simulink model "Battery_charge_discharge_FSBB_DCDC"  (R2022b)
settings: Solver=ode23tb  StartTime=0.0  StopTime=1.5  RelTol=1e-3  EnableMultiTasking=on
values from neighbouring files (symbols this model uses):
  time_step = 1 / wave_freq    (= 1.11111111111e-05)    [Battery_charge_discharge_FSBB_param_init.m]
undefined symbols (not defined in the file or in its folder): Ion, Lithium
libraries: spsTriangleGeneratorLib x13, spsSeriesRLCBranchLib x9, slpidlib x9, spsVoltageMeasurementLib x5, spsCurrentMeasurementLib x4, spsIGBTDiodeLib x4, spsBatteryLib x2, spsIdealSwitchLib x2, spsDCVoltageSourceLib x2, spsControlledVoltageSourceLib x1, spspowerguiLib x1
(part 1 of 2)
settings Model: Creator=Lei  LastModifiedBy=Loki
settings SolverCC: AlgebraicLoopSolver=TrustRegion
settings DataIOCC: LimitDataPoints=on  SaveFormat=Array  ReturnWorkspaceOutputs=off
settings OptimizationCC: LifeSpan=inf
settings DebuggingCC: SolverPrmCheckMsg=warning  UnconnectedInputMsg=warning  UnconnectedOutputMsg=warning  UnconnectedLineMsg=warning  SFUnexpectedBacktrackingDiag=warning  SFNoUnconditionalDefaultTransitionDiag=warning  SFExecutionAtInitializationDiag=none  SFMachineParentedDataDiag=warning  ArithmeticOperatorsInVariantConditions=warning
settings HardwareCC: ProdBitPerPointer=32  ProdBitPerSizeT=32  ProdBitPerPtrDiffT=32  ProdLargestAtomicFloat=None  ProdIntDivRoundTo=Undefined  ProdEndianess=Unspecified  ProdWordSize=32  ProdHWDeviceType=32-bit Generic
settings ModelReferenceCC: EnableRefExpFcnMdlSchedulingChecks=on  PropagateSignalLabelsOutOfModel=off
settings SFSimCC: SimUseLocalCustomCode=off  CustomCodeUndefinedFunction=UseInterfaceOnly
settings RTWCC: RTWUseLocalCustomCode=off
settings CodeAppCC: StateflowObjectComments=on
settings GRTTargetCC: TargetLangStandard=C89/C90 (ANSI)
settings ConfigComp: CovMetricSettings=dw  CovSaveCumulativeToWorkspaceVar=on  CovSaveSingleToWorkspaceVar=on  CovExternalEMLEnable=off  CovSFcnEnable=off
settings SimscapeCC: SimscapeNormalizeSystem=off

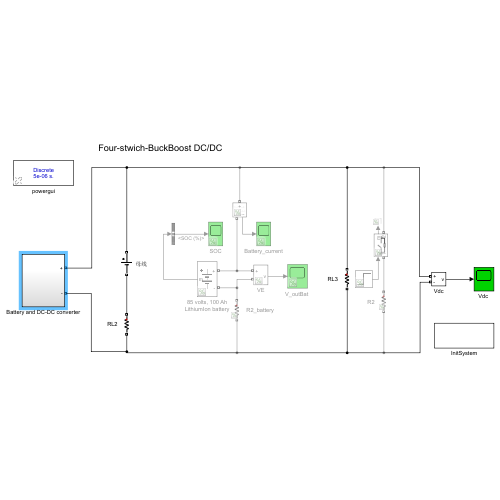
[thumbnail: Simulink's stored preview of the top-level diagram]
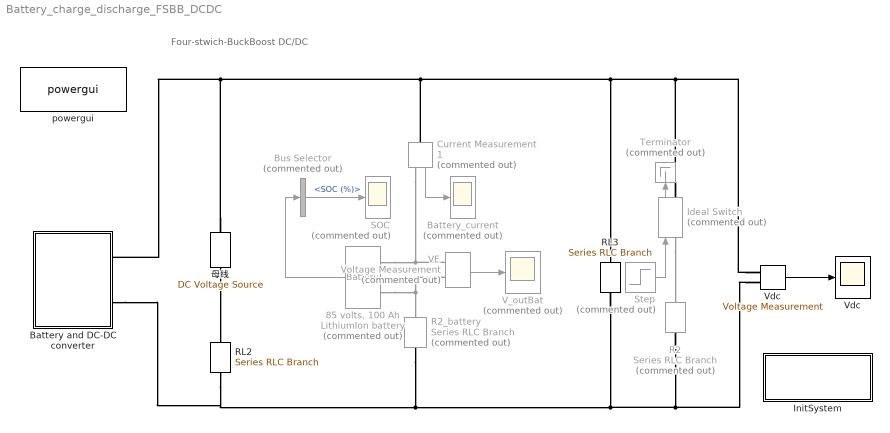
== system Battery_charge_discharge_FSBB_DCDC ==
  note: Four-stwich-BuckBoost DC/DC
  "85 volts, 100 Ah LithiumIon battery " : spsBatteryLib/Battery  Commented=on  BatType=Lithium-Ion  ShowTempParam=off  ThermalPreset=no  ShowAgeParam=off  NomV=85  NomQ=100  SOC=90  Batt_Tr=30  PresetModel=off  MaxQ=107.6923  MinV=83.2  FullV=115.2  Dis_rate=20  R=0.0085  Normal_OP=96.1538  expZone="[92.2034           20]"  current=[6.5 13 32.5]  Units=Time  Tci=20  NomT=20  T2=-30  MaxQ2=4.8  FullV2=7.1  Normal_OP2=5.655  expZone2="[6.58           1]"  Rca=0.6  ti=2000  Dp=0  Neq0=0  Tsim=1e6  Ta1=25  Qeol=5.4*0.9  Reol=0.013333*1.2  Char_age=[2.3478, 3]  Dis_age=[2.3478, 10]  N1=1500  N2=10500  N3=1000  N4=1400  Ta2=45  N5=950
      settings: LibrarySourceBlock=electricdrivelib/Extra Sources/Battery
  Battery and DC-DC converter : Subsystem
  Battery_current : Scope  Commented=on
  Bus Selector : BusSelector  Commented=on  OutputSignals=SOC (%)
  Current Measurement1 : spsCurrentMeasurementLib/Current Measurement  Commented=on  PhasorSimulation=off  OutputType=Complex  PSBequivalent=0
  Ideal Switch : spsIdealSwitchLib/Ideal Switch  Commented=on  Ron=0.001  Lon=0  IC=0  Rs=1e5  Cs=inf  Measurements=on
  InitSystem : Subsystem
      settings: OpenFcn=Battery_charge_discharge_FSBB_param_init
  R2 : spsSeriesRLCBranchLib/Series RLC Branch  Commented=on  LConnTagsString=__new0  RConnTagsString=__new0  BranchType=R  Resistance=6  Inductance=1e-3  SetiL0=off  InitialCurrent=0  Capacitance=1e-6  Setx0=off  InitialVoltage=0  Measurements=None
  R2_battery : spsSeriesRLCBranchLib/Series RLC Branch  Commented=on  LConnTagsString=__new0  RConnTagsString=__new0  BranchType=R  Resistance=0.1  Inductance=1e-3  SetiL0=off  InitialCurrent=0  Capacitance=1440e-6  Setx0=off  InitialVoltage=80  Measurements=None
  RL2 : spsSeriesRLCBranchLib/Series RLC Branch  LConnTagsString=__new0  RConnTagsString=__new0  BranchType=R  Resistance=0.1  Inductance=1e-3  SetiL0=off  InitialCurrent=0  Capacitance=1e-6  Setx0=off  InitialVoltage=0  Measurements=None
  RL3 : spsSeriesRLCBranchLib/Series RLC Branch  LConnTagsString=__new0  RConnTagsString=__new0  BranchType=R  Resistance=6  Inductance=1e-3  SetiL0=off  InitialCurrent=0  Capacitance=1e-6  Setx0=off  InitialVoltage=0  Measurements=None
  SOC : Scope  Commented=on
  Step : Step  Commented=on  Time=0.3  After=3  SampleTime=0
  Terminator : Terminator  Commented=on
  VE : spsVoltageMeasurementLib/Voltage Measurement  Commented=on  PhasorSimulation=off  OutputType=Complex  PSBequivalent=0
  "V_outBat " : Scope  Commented=on
  Vdc : spsVoltageMeasurementLib/Voltage Measurement  PhasorSimulation=off  OutputType=Complex  PSBequivalent=0
  "Vdc " : Scope
  powergui : spspowerguiLib/powergui  Priority=1  SimulationMode=Discrete  SampleTime=5e-6  frequency=60  Iterations=50  frequencyindice=0  Pbase=100e6  ErrMax=1e-4  UnitsV=kV  UnitsW=MW  buscounter=0  FunctionMessages=off  echomessages=off  EnableUseOfTLC=off  CurrentSourceSwitches=off  DisableSnubberDevices=off  DisableRonSwitches=off  DisableVfSwitches=off  DisplayEquations=off  AutomaticDiscreteSolvers=off  SolverType=Tustin/Backward Euler (TBE)  Interpol=off  ExternalGateDelay=off  methode=off  Ts=100  x0status=blocks  SPID=off  SwTol=0  HookPort=off  NonlinearTolerance=1e-4  nMaxIteration=100  ContinueOnMaxIteration=off  RestoreLinks=warning  ResistiveCurrentMeasurement=off  Frange=[0:2:500]  Ylog=off  Xlog=on  ShowGrid=off  save=off  variable=ZData  structure=0  ZoomFFT=off  StartTime=0.0  cycles=1  DisplayStyle=1  fundamental=60  FreqAxis=off  MaxFrequency=1000  frequencyindicesteady=1  RmsSteady=1  display=off
  "母线  " : spsDCVoltageSourceLib/DC Voltage Source  Amplitude=104  Measurements=None
  wires:
  Vdc/1 -> "Vdc "/1
  Step/1 -> Ideal Switch/1
  Ideal Switch/1 -> Terminator/1
  Bus Selector/1 -> SOC/1  "<SOC (%)>"
  "85 volts, 100 Ah LithiumIon battery "/1 -> Bus Selector/1
  Current Measurement1/1 -> Battery_current/1
  VE/1 -> "V_outBat "/1
  connections:
  Vdc/LConn1 -- Ideal Switch/RConn1 -- Current Measurement1/LConn1 -- "母线  "/RConn1 -- Battery and DC-DC converter/RConn1 -- RL3/LConn1
  Vdc/LConn2 -- R2/RConn1 -- RL3/RConn1 -- RL2/RConn1 -- Battery and DC-DC converter/RConn2 -- R2_battery/RConn1
  "母线  "/LConn1 -- RL2/LConn1
  Ideal Switch/LConn1 -- R2/LConn1
  VE/LConn2 -- "85 volts, 100 Ah LithiumIon battery "/LConn2 -- R2_battery/LConn1
  VE/LConn1 -- Current Measurement1/RConn1 -- "85 volts, 100 Ah LithiumIon battery "/LConn1

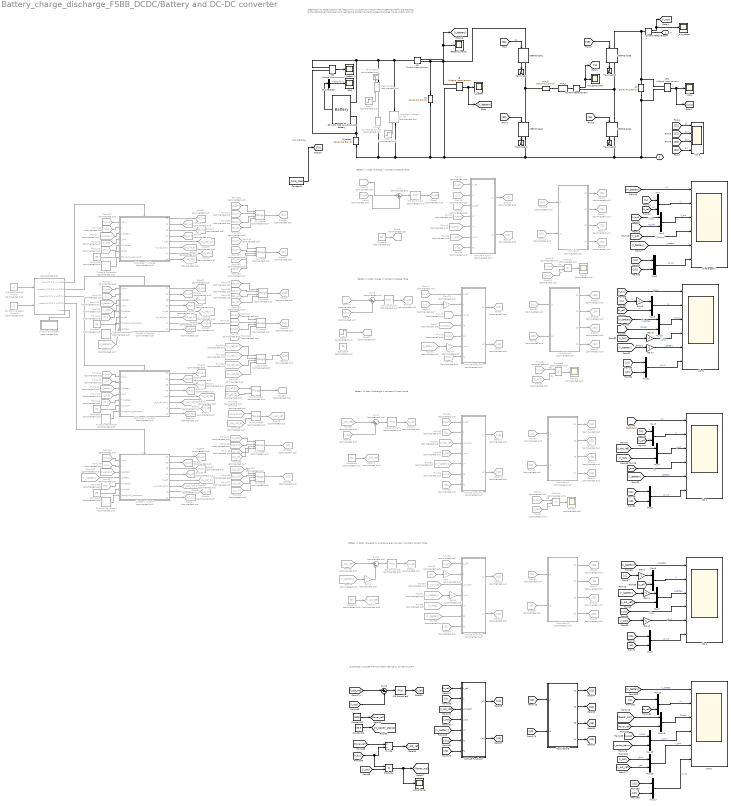
== system Battery_charge_discharge_FSBB_DCDC/Battery and DC-DC converter ==
  note: Discharge in Constant Power Mode: realize by constant current
  note: Battery in dcdc , charged by outside energy source in constant Current Mode
  note: Battery in dcdc ,discharge in constant Current Mode
  note: Battery in dcdc, dicharge in constant Voltage Mode
  note: 和开关频率同步
  note: FSBB Passivity Based Control
      | ref: https://www.youtube.com/watch?v=5YT7cERlMrg
      | Modify the topology to the Gosspower hardware's
      | and realize the constant current/voltage discharge mode.
      | Author LokiXun
  note: Battery in dcdc, charge in constant Voltage Mode
  "85 volts, 100 Ah LithiumIon battery " : spsBatteryLib/Battery  BatType=Lithium-Ion  ShowTempParam=off  ThermalPreset=no  ShowAgeParam=off  NomV=85  NomQ=100  SOC=80  Batt_Tr=30  PresetModel=off  MaxQ=107.6923  MinV=83.2  FullV=115.2  Dis_rate=20  R=0.0085  Normal_OP=96.1538  expZone="[92.2034           20]"  current=[6.5 13 32.5]  Units=Time  Tci=20  NomT=20  T2=-30  MaxQ2=4.8  FullV2=7.1  Normal_OP2=5.655  expZone2="[6.58           1]"  Rca=0.6  ti=2000  Dp=0  Neq0=0  Tsim=1e6  Ta1=25  Qeol=5.4*0.9  Reol=0.013333*1.2  Char_age=[2.3478, 3]  Dis_age=[2.3478, 10]  N1=1500  N2=10500  N3=1000  N4=1400  Ta2=45  N5=950
      settings: LibrarySourceBlock=electricdrivelib/Extra Sources/Battery
  ActualPower : Scope
  BatteryCurrent1 : Scope
  Bus Selector : BusSelector  OutputSignals=SOC (%)
  C1 : spsSeriesRLCBranchLib/Series RLC Branch  LConnTagsString=__new0  RConnTagsString=__new0  BranchType=C  Resistance=0.01  Inductance=1e-3  SetiL0=off  InitialCurrent=0  Capacitance=1440e-6  Setx0=off  InitialVoltage=80  Measurements=None
  C2 : spsSeriesRLCBranchLib/Series RLC Branch  LConnTagsString=__new0  RConnTagsString=__new0  BranchType=C  Resistance=5  Inductance=1e-3  SetiL0=off  InitialCurrent=0  Capacitance=1440e-6  Setx0=off  InitialVoltage=80  Measurements=None
  Charge + Current : Subsystem  Commented=on  TreatAsAtomicUnit=on
  Charge + Voltage : Subsystem  Commented=on  TreatAsAtomicUnit=on
  Charge/Discharge Mode : Constant  Commented=on  Value=0
  Constant{,4,6..7} (4 alike) : Constant  Commented=on  Value=96
  Constant Voltage / Current : Constant  Commented=on
  Constant1 : Constant  Value=time_step
  Constant10 : Constant  Value=3000
  Constant11 : Constant  Value=103.5
  Constant2 : Constant  Commented=on  Value=30
  Constant3 : Constant  Commented=on  Value=29
  Constant8 : Constant  Commented=on  Value=29
  Constant9 : Constant  Commented=on  Value=29
  Controlled Voltage Source : spsControlledVoltageSourceLib/Controlled Voltage Source  Commented=on  Initialize=on  Source_Type=DC  Amplitude=103  Phase=0  Frequency=0  Measurements=None
  Current Measurement : spsCurrentMeasurementLib/Current Measurement  PhasorSimulation=off  OutputType=Complex  PSBequivalent=0
  Current Measurement1 : spsCurrentMeasurementLib/Current Measurement  PhasorSimulation=off  OutputType=Complex  PSBequivalent=0
  Discharge + Current : Subsystem  Commented=on  TreatAsAtomicUnit=on
  Discharge + Voltage : Subsystem  Commented=on  TreatAsAtomicUnit=on
  Discharge+V : Scope  NumInputPorts=6
  Divide : Product  Inputs=*/
  From{10,24,30,32,116,121,143,156} (8 alike) : From  Commented=on  GotoTag=iL
  From{11..12,70,75} (4 alike) : From  Commented=on  GotoTag=VC_ref
  From{8,13,28,41,52..53,76,92,94,115,120,142,155} (13 alike) : From  Commented=on  GotoTag=V_bus
  From{14,33,59,77,117,122,144,157} (8 alike) : From  Commented=on  GotoTag=V_battery
  From{29,31,42,55,88,96,118,123,145} (9 alike) : From  Commented=on  GotoTag=i_out
  From{18,35,54,78,119,124,146,159} (8 alike) : From  Commented=on  GotoTag=Ts
  From125 : From  Commented=on  GotoTag=S1_DV
  From126 : From  Commented=on  GotoTag=S2_DV
  From127 : From  Commented=on  GotoTag=S1_CV
  From128 : From  Commented=on  GotoTag=S2_CV
  From129 : From  Commented=on  GotoTag=S3_DV
  From130 : From  Commented=on  GotoTag=S3_CV
  From131 : From  Commented=on  GotoTag=S4_CV
  From132 : From  Commented=on  GotoTag=S4_DV
  From133 : From  Commented=on  GotoTag=iL_ref_CV
  From134 : From  Commented=on  GotoTag=iL_ref_DV
  From135 : From  Commented=on  GotoTag=VC_ref_CV
  From136 : From  Commented=on  GotoTag=VC_ref_DV
  From137 : From  Commented=on  GotoTag=u1_DV
  From138 : From  Commented=on  GotoTag=u1_CV
  From139 : From  Commented=on  GotoTag=u2_DV
  From140 : From  Commented=on  GotoTag=u2_CV
  From{34,74,95,141,160} (5 alike) : From  Commented=on  GotoTag=i_battery
  From147 : From  Commented=on  GotoTag=u2_DI
  From148 : From  Commented=on  GotoTag=u1_DI
  From149 : From  Commented=on  GotoTag=i_out_ref_DI
  From150 : From  Commented=on  GotoTag=iL_ref_DI
  From151 : From  Commented=on  GotoTag=S4_DI
  From152 : From  Commented=on  GotoTag=S3_DI
  From153 : From  Commented=on  GotoTag=S2_DI
  From154 : From  Commented=on  GotoTag=S1_DI
  From158 : From  Commented=on  GotoTag=i_out_ref_CI
  From{16,39,61,80} (4 alike) : From  Commented=on  GotoTag=u1
  From161 : From  Commented=on  GotoTag=S1_CI
  From162 : From  Commented=on  GotoTag=S2_CI
  From163 : From  Commented=on  GotoTag=S3_CI
  From164 : From  Commented=on  GotoTag=S4_CI
  From165 : From  Commented=on  GotoTag=iL_ref_CI
  From166 : From  Commented=on  GotoTag=u1_CI
  From167 : From  Commented=on  GotoTag=u2_CI
  From{17,40,62,81} (4 alike) : From  Commented=on  GotoTag=u2
  From{9,36,56,79} (4 alike) : From  Commented=on  GotoTag=iL_ref
  From{37..38,57..58} (4 alike) : From  Commented=on  GotoTag=i_out_ref
  Gain{,2..3,6,10} (5 alike) : Gain  Commented=on  Gain=-1
  Gain{1,4..5,7..9} (6 alike) : Gain  Gain=-1
  Goto{10,21,28..29,58} (5 alike) : Goto  Commented=on  GotoTag=S4
  Goto{11,22,30,33,56} (5 alike) : Goto  Commented=on  GotoTag=S2
  Goto{6,12,15,17,61} (5 alike) : Goto  Commented=on  GotoTag=u1
  Goto{7,14,18,25,62} (5 alike) : Goto  Commented=on  GotoTag=u2
  Goto19 : Goto  Commented=on  GotoTag=i_out_ref
  Goto{2,20,27,36,60} (5 alike) : Goto  Commented=on  GotoTag=iL_ref
  Goto{8,23,31,40,59} (5 alike) : Goto  Commented=on  GotoTag=S1
  Goto{9,24,32,41,57} (5 alike) : Goto  Commented=on  GotoTag=S3
  Goto26 : Goto  Commented=on  GotoTag=i_out_ref
  Goto37 : Goto  Commented=on  GotoTag=VC_ref
  Goto47 : Goto  Commented=on  GotoTag=VC_ref_DV
  Goto48 : Goto  Commented=on  GotoTag=S2_DV
  Goto49 : Goto  Commented=on  GotoTag=S3_DV
  Goto5 : Goto  Commented=on  GotoTag=VC_ref
  Goto50 : Goto  Commented=on  GotoTag=S4_DV
  Goto51 : Goto  Commented=on  GotoTag=S1_DV
  Goto52 : Goto  Commented=on  GotoTag=iL_ref_DV
  Goto53 : Goto  Commented=on  GotoTag=u1_DV
  Goto54 : Goto  Commented=on  GotoTag=u2_DV
  Goto55 : Goto  Commented=on  GotoTag=VC_ref
  Goto63 : Goto  Commented=on  GotoTag=VC_ref_CV
  Goto64 : Goto  Commented=on  GotoTag=S2_CV
  Goto65 : Goto  Commented=on  GotoTag=S3_CV
  Goto66 : Goto  Commented=on  GotoTag=S4_CV
  Goto67 : Goto  Commented=on  GotoTag=S1_CV
  Goto68 : Goto  Commented=on  GotoTag=iL_ref_CV
  Goto69 : Goto  Commented=on  GotoTag=u1_CV
  Goto70 : Goto  Commented=on  GotoTag=u2_CV
  Goto71 : Goto  Commented=on  GotoTag=i_out_ref_DI
  Goto72 : Goto  Commented=on  GotoTag=S2_DI
  Goto73 : Goto  Commented=on  GotoTag=S3_DI
  Goto74 : Goto  Commented=on  GotoTag=S4_DI
  Goto75 : Goto  Commented=on  GotoTag=S1_DI
  Goto76 : Goto  Commented=on  GotoTag=iL_ref_DI
  Goto77 : Goto  Commented=on  GotoTag=u1_DI
  Goto78 : Goto  Commented=on  GotoTag=u2_DI
  Goto79 : Goto  Commented=on  GotoTag=i_out_ref
  Goto80 : Goto  Commented=on  GotoTag=i_out_ref_CI
  Goto81 : Goto  Commented=on  GotoTag=S2_CI
  Goto82 : Goto  Commented=on  GotoTag=S3_CI
  Goto83 : Goto  Commented=on  GotoTag=S4_CI
  Goto84 : Goto  Commented=on  GotoTag=S1_CI
  Goto85 : Goto  Commented=on  GotoTag=iL_ref_CI
  Goto86 : Goto  Commented=on  GotoTag=u1_CI
  Goto87 : Goto  Commented=on  GotoTag=u2_CI
  IGBT/Diode{1..4} (4 alike) : spsIGBTDiodeLib/IGBT//Diode  Ron=1e-3  Rs=1e5  Cs=inf  Measurements=on
  IL6 : spsCurrentMeasurementLib/Current Measurement  PhasorSimulation=off  OutputType=Complex  PSBequivalent=0
  I_bus_scope : Scope
  Ideal Switch : spsIdealSwitchLib/Ideal Switch  Commented=on  Ron=0.001  Lon=0  IC=0  Rs=1e5  Cs=inf  Measurements=on
  If : If  Commented=on  NumInputs=2  IfExpression=u1 == 1 & u2 ==0  ElseIfExpressions=u1 == 0 & u2 ==0, u1==1 & u2==1, u1==0 & u2==1
  If Action Subsystem : Subsystem  Commented=on  TreatAsAtomicUnit=on
  InductorCurrent : Scope
  MATLAB Function : MATLAB Function  Commented=on  TreatAsAtomicUnit=on
  MATLAB Function1 : MATLAB Function  Commented=on  TreatAsAtomicUnit=on
  MATLAB Function2 : MATLAB Function  Commented=on  TreatAsAtomicUnit=on
  MATLAB Function3 : MATLAB Function  Commented=on  TreatAsAtomicUnit=on
  MATLAB Function5 : MATLAB Function  TreatAsAtomicUnit=on
  Modulation : Subsystem  Commented=on
  Modulation1 : Subsystem  Commented=on
  Modulation2 : Subsystem  Commented=on
  Modulation3 : Subsystem  Commented=on
  Modulation5 : Subsystem
  Mux{,1..11,15..19} (17 alike) : Mux  Inputs=2
  PID Controller{1..4} (4 alike) : slpidlib/PID Controller  Commented=on  Controller=PI  Form=Parallel  TimeDomain=Continuous-time  UseExternalTs=off  SampleTime=-1  IntegratorMethod=Forward Euler  FilterMethod=Forward Euler  ControllerParametersSource=internal  P=15  I=1000  UseKiTs=on  D=0  N=100  UseFilter=on  TunerSelectOption=Transfer Function Based (PID Tuner App)  InitialConditionSource=internal  InitialConditionForIntegrator=0  InitialConditionForFilter=0  DifferentiatorICPrevScaledInput=0  ExternalReset=none  TrackingMode=off  Kt=1  LimitOutput=on  SatLimitsSource=internal  UpperSaturationLimit=50  LowerSaturationLimit=-10  LinearizeAsGain=on  AntiWindupMode=none  Kb=1  LimitIntegrator=off  UpperIntegratorSaturationLimit=inf  LowerIntegratorSaturationLimit=-inf  POutMin=[]  POutMax=[]  IOutMin=[]  IOutMax=[]  DOutMin=[]  DOutMax=[]  NOutMin=[]  NOutMax=[]  SumOutMin=[]  SumOutMax=[]  SaturationOutMin=[]  SaturationOutMax=[]  PParamMin=[]  PParamMax=[]  IParamMin=[]  IParamMax=[]  DParamMin=[]  DParamMax=[]  NParamMin=[]  NParamMax=[]  KbParamMin=[]  KbParamMax=[]  KtParamMin=[]  KtParamMax=[]  KbOutMin=[]  KbOutMax=[]  KtOutMin=[]  KtOutMax=[]  IntegratorOutMin=[]  IntegratorOutMax=[]  FilterOutMin=[]  FilterOutMax=[]  SumI1OutMin=[]  SumI1OutMax=[]  SumI2OutMin=[]  SumI2OutMax=[]  SumI3OutMin=[]  SumI3OutMax=[]  SumI4OutMin=[]  SumI4OutMax=[]  SumDOutMin=[]  SumDOutMax=[]  DifferentiatorOutMin=[]  DifferentiatorOutMax=[]  FilterDiffOutCoefMin=[]  FilterDiffOutCoefMax=[]  ReciprocalOutMin=[]  ReciprocalOutMax=[]  SumDenOutMin=[]  SumDenOutMax=[]  SumNumOutMin=[]  SumNumOutMax=[]  DivideOutMin=[]  DivideOutMax=[]  UdiffTsProdOutMin=[]  UdiffTsProdOutMax=[]  NTsProdOutMin=[]  NTsProdOutMax=[]  UintegralTsProdOutMin=[]  UintegralTsProdOutMax=[]  UngainTsProdOutMin=[]  UngainTsProdOutMax=[]  ClampingZeroOutDataTypeStr=Inherit: Inherit via back propagation  ClampingZeroOutMin=[]  ClampingZeroOutMax=[]  FilterDenConstantOutDataTypeStr=Inherit: Inherit via back propagation  FilterDenConstantOutMin=[]  FilterDenConstantOutMax=[]  PCopyOutDataTypeStr=Inherit: Inherit via back propagation  PCopyOutMin=[]  PCopyOutMax=[]  NCopyOutDataTypeStr=Inherit: Inherit via back propagation  NCopyOutMin=[]  NCopyOutMax=[]  IntegratorContinuousStateAttributes=''  IntegratorStateMustResolveToSignalObject=off  IntegratorRTWStateStorageClass=Auto  FilterContinuousStateAttributes=''  FilterStateMustResolveToSignalObject=off  FilterRTWStateStorageClass=Auto  ParallelPVariant=InternalParameters  IdealPVariant=Disabled  IVariant=InternalParameters  DVariant=Disabled  IntegratorVariant=Continuous  SatVariant=Enabled  AWVariant=Passthrough  PCopyVariant=Disabled  TRVariant=Disabled  FdbkBlocksVariant=Forward  IdealPFdbkVariant=Disabled  SatFdbkVariant=Disabled  DerivativeFilterVariant=Disabled  NVariant=Disabled  NCopyVariant=Disabled_SignalSpec  FilterICVariant=Disabled  IntegratorICVariant=InternalICs  ExternalResetVariant=Disabled  TRSumVariant=Passthrough  SumFdbkVariant=Disabled  SumVariant=Sum_PI  TsampFilterVariant=InternalTs  TsampNgainVariant=Passthrough  TsampIntegralVariant=Passthrough  ExternalSaturationOutDataTypeStr=Inherit: Same as second input
  PID Controller6 : slpidlib/PID Controller  Controller=PI  Form=Parallel  TimeDomain=Continuous-time  UseExternalTs=off  SampleTime=-1  IntegratorMethod=Forward Euler  FilterMethod=Forward Euler  ControllerParametersSource=internal  P=15  I=1000  UseKiTs=on  D=0  N=100  UseFilter=on  TunerSelectOption=Transfer Function Based (PID Tuner App)  InitialConditionSource=internal  InitialConditionForIntegrator=0  InitialConditionForFilter=0  DifferentiatorICPrevScaledInput=0  ExternalReset=none  TrackingMode=off  Kt=1  LimitOutput=on  SatLimitsSource=internal  UpperSaturationLimit=50  LowerSaturationLimit=-10  LinearizeAsGain=on  AntiWindupMode=none  Kb=1  LimitIntegrator=off  UpperIntegratorSaturationLimit=inf  LowerIntegratorSaturationLimit=-inf  POutMin=[]  POutMax=[]  IOutMin=[]  IOutMax=[]  DOutMin=[]  DOutMax=[]  NOutMin=[]  NOutMax=[]  SumOutMin=[]  SumOutMax=[]  SaturationOutMin=[]  SaturationOutMax=[]  PParamMin=[]  PParamMax=[]  IParamMin=[]  IParamMax=[]  DParamMin=[]  DParamMax=[]  NParamMin=[]  NParamMax=[]  KbParamMin=[]  KbParamMax=[]  KtParamMin=[]  KtParamMax=[]  KbOutMin=[]  KbOutMax=[]  KtOutMin=[]  KtOutMax=[]  IntegratorOutMin=[]  IntegratorOutMax=[]  FilterOutMin=[]  FilterOutMax=[]  SumI1OutMin=[]  SumI1OutMax=[]  SumI2OutMin=[]  SumI2OutMax=[]  SumI3OutMin=[]  SumI3OutMax=[]  SumI4OutMin=[]  SumI4OutMax=[]  SumDOutMin=[]  SumDOutMax=[]  DifferentiatorOutMin=[]  DifferentiatorOutMax=[]  FilterDiffOutCoefMin=[]  FilterDiffOutCoefMax=[]  ReciprocalOutMin=[]  ReciprocalOutMax=[]  SumDenOutMin=[]  SumDenOutMax=[]  SumNumOutMin=[]  SumNumOutMax=[]  DivideOutMin=[]  DivideOutMax=[]  UdiffTsProdOutMin=[]  UdiffTsProdOutMax=[]  NTsProdOutMin=[]  NTsProdOutMax=[]  UintegralTsProdOutMin=[]  UintegralTsProdOutMax=[]  UngainTsProdOutMin=[]  UngainTsProdOutMax=[]  ClampingZeroOutDataTypeStr=Inherit: Inherit via back propagation  ClampingZeroOutMin=[]  ClampingZeroOutMax=[]  FilterDenConstantOutDataTypeStr=Inherit: Inherit via back propagation  FilterDenConstantOutMin=[]  FilterDenConstantOutMax=[]  PCopyOutDataTypeStr=Inherit: Inherit via back propagation  PCopyOutMin=[]  PCopyOutMax=[]  NCopyOutDataTypeStr=Inherit: Inherit via back propagation  NCopyOutMin=[]  NCopyOutMax=[]  IntegratorContinuousStateAttributes=''  IntegratorStateMustResolveToSignalObject=off  IntegratorRTWStateStorageClass=Auto  FilterContinuousStateAttributes=''  FilterStateMustResolveToSignalObject=off  FilterRTWStateStorageClass=Auto  ParallelPVariant=InternalParameters  IdealPVariant=Disabled  IVariant=InternalParameters  DVariant=Disabled  IntegratorVariant=Continuous  SatVariant=Enabled  AWVariant=Passthrough  PCopyVariant=Disabled  TRVariant=Disabled  FdbkBlocksVariant=Forward  IdealPFdbkVariant=Disabled  SatFdbkVariant=Disabled  DerivativeFilterVariant=Disabled  NVariant=Disabled  NCopyVariant=Disabled_SignalSpec  FilterICVariant=Disabled  IntegratorICVariant=InternalICs  ExternalResetVariant=Disabled  TRSumVariant=Passthrough  SumFdbkVariant=Disabled  SumVariant=Sum_PI  TsampFilterVariant=InternalTs  TsampNgainVariant=Passthrough  TsampIntegralVariant=Passthrough  ExternalSaturationOutDataTypeStr=Inherit: Same as second input
  Power : Scope  Commented=on
  Power1 : Scope  Commented=on
  Power3 : Scope  Commented=on
  Product : Product  Commented=on
  Product1 : Product  Commented=on
  Product3 : Product  Commented=on
  Product4 : Product
  R_battery : spsSeriesRLCBranchLib/Series RLC Branch  LConnTagsString=__new0  RConnTagsString=__new0  BranchType=R  Resistance=0.1  Inductance=1e-3  SetiL0=off  InitialCurrent=0  Capacitance=1440e-6  Setx0=off  InitialVoltage=80  Measurements=None
  S1_merge : Merge  Commented=on  Inputs=4  InitialOutput=[0]
  S2_merge : Merge  Commented=on  Inputs=4  InitialOutput=[0]
  S3_merge : Merge  Commented=on  Inputs=4  InitialOutput=[0]
  S4_merge : Merge  Commented=on  Inputs=4  InitialOutput=[0]
  SOC : Scope
  Step : Step  Commented=on  Time=0.7  Before=103  After=93  SampleTime=0
  Step1 : Step  Commented=on  Time=0.002  Before=1  After=0  SampleTime=0
  Step2 : Step  Commented=on  Time=0.4  Before=30  After=40  SampleTime=0
  Sum{,1..3} (4 alike) : Sum  Commented=on  Inputs=|+-
  Sum5 : Sum  Inputs=|+-
  Terminator{,1..3} (4 alike) : Terminator
  Terminator4 : Terminator  Commented=on
  Triangle Generator{,1..3} (4 alike) : spsTriangleGeneratorLib/Triangle Generator  Commented=on  Freq=wave_freq  Phase=0  Ts=0
  VE : spsVoltageMeasurementLib/Voltage Measurement  PhasorSimulation=off  OutputType=Complex  PSBequivalent=0
  VE1 : spsVoltageMeasurementLib/Voltage Measurement  PhasorSimulation=off  OutputType=Complex  PSBequivalent=0
  VE2 : spsVoltageMeasurementLib/Voltage Measurement  PhasorSimulation=off  OutputType=Complex  PSBequivalent=0
  "V_battery " : Scope
  V_battery 1 : Scope
  V_bus : Scope
  Vc_ref_merge : Merge  Commented=on  InitialOutput=[0]
  Vc_ref_merge1 : Merge  Commented=on  InitialOutput=[0]
  Vdc 1 : Scope  NumInputPorts=4
  Vdc {2..5} (4 alike) : Scope  NumInputPorts=6
  iL_ref_merge : Merge  Commented=on  Inputs=4  InitialOutput=[0]
  "init_bat  " : spsDCVoltageSourceLib/DC Voltage Source  Commented=on  Amplitude=93.5  Measurements=None
  mid_L : spsSeriesRLCBranchLib/Series RLC Branch  LConnTagsString=__new0  RConnTagsString=__new0  BranchType=L  Resistance=1.0  Inductance=20e-6  SetiL0=off  InitialCurrent=0  Capacitance=1.0  Setx0=off  InitialVoltage=0  Measurements=None
  mid_R : spsSeriesRLCBranchLib/Series RLC Branch  LConnTagsString=__new0  RConnTagsString=__new0  BranchType=R  Resistance=0.004  Inductance=1e-3  SetiL0=off  InitialCurrent=0  Capacitance=1e-3  Setx0=off  InitialVoltage=80  Measurements=None
  u1_merge1 : Merge  Commented=on  Inputs=4  InitialOutput=[0]
  u2_merge : Merge  Commented=on  Inputs=4  InitialOutput=[0]
  + : PMIOPort  Tag=PMCPort  Side=Right
  - : PMIOPort  Tag=PMCPort  Port=2  Side=Right
  wires:
  VE/1 -> [V_battery], "V_battery "/1
  Bus Selector/1 -> SOC/1  "<SOC (%)>"
  "85 volts, 100 Ah LithiumIon battery "/1 -> Bus Selector/1
  [S2] -> IGBT/Diode2/1
  [S1] -> IGBT/Diode1/1  "S1"
  [S1] -> Vdc 1/1  "S1"
  [S2] -> Vdc 1/2  "S2"
  [S3] -> Vdc 1/3  "S3"
  [S4] -> Vdc 1/4  "S4"
  Current Measurement/1 -> [iL], InductorCurrent/1
  [S3] -> IGBT/Diode3/1
  [S4] -> IGBT/Diode4/1
  Sum/1 -> PID Controller2/1
  PID Controller2/1 -> Goto2/1
  Current Measurement1/1 -> [i_out], I_bus_scope/1
  From9/1 -> MATLAB Function/1(iL_ref)
  From10/1 -> MATLAB Function/2(iL)
  From12/1 -> MATLAB Function/3(vc_ref)
  From13/1 -> MATLAB Function/4(vc)
  From14/1 -> MATLAB Function/5(vin)
  From18/1 -> MATLAB Function/7(Ts)
  From96/1 -> MATLAB Function/6(i_out)
  From16/1 -> Modulation/1(u1)
  From17/1 -> Modulation/2(u2)
  Modulation/1(S1) -> Goto8/1
  Modulation/3(S3) -> Goto9/1
  Modulation/4(S4) -> Goto10/1
  Modulation/2(S2) -> Goto11/1
  Constant1/1 -> [Ts]
  [V_battery] -> Discharge+V/1  "Vin"
  Mux/1 -> Discharge+V/2  "iL"
  [iL_ref] -> Mux/2  "iL*"
  [iL] -> Mux/1  "iL"
  [V_bus] -> Mux1/1  "V_bus"
  [VC_ref] -> Mux1/2  "VC_ref"
  Mux1/1 -> Discharge+V/3  "V_out"
  Mux2/1 -> Discharge+V/6  "u1,u2"
  [u1] -> Mux2/1
  [u2] -> Mux2/2
  IGBT/Diode1/1 -> Terminator/1
  IGBT/Diode2/1 -> Terminator1/1
  IGBT/Diode4/1 -> Terminator2/1
  IGBT/Diode3/1 -> Terminator3/1
  VE1/1 -> [V_bus], V_bus/1
  MATLAB Function/2(u2) -> Goto14/1
  MATLAB Function/1(u1) -> Goto12/1
  [i_out] -> Discharge+V/4  "i_output"
  [i_battery] -> Discharge+V/5  "i_battery"
  From11/1 -> Sum/1
  From28/1 -> Product/1  "Vc"
  From29/1 -> Product/2  "io"
  Product/1 -> Power/1
  From8/1 -> Sum/2
  From30/1 -> MATLAB Function1/2(iL)
  From55/1 -> MATLAB Function1/4(i_out)
  From36/1 -> MATLAB Function1/1(iL_ref)
  From37/1 -> MATLAB Function1/3(i_out_ref)
  From33/1 -> MATLAB Function1/5(vin)
  MATLAB Function1/1(u1) -> Goto17/1
  From35/1 -> MATLAB Function1/7(Ts)
  MATLAB Function1/2(u2) -> Goto18/1
  Constant3/1 -> Goto19/1
  From38/1 -> Sum1/1
  Sum1/1 -> PID Controller1/1
  From31/1 -> Sum1/2
  PID Controller1/1 -> Goto20/1
  From41/1 -> Product1/1  "Vc"
  Modulation1/4(S4) -> Goto21/1
  Modulation1/1(S1) -> Goto23/1
  From40/1 -> Modulation1/2(u2)
  Modulation1/2(S2) -> Goto22/1
  Modulation1/3(S3) -> Goto24/1
  From42/1 -> Product1/2  "io"
  From39/1 -> Modulation1/1(u1)
  Product1/1 -> Power1/1
  [iL_ref] -> Mux3/2  "iL*"
  [u1] -> Mux5/1
  Mux5/1 -> Vdc 2/6  "u1,u2"
  [V_battery] -> Vdc 2/1  "Vin"
  [i_battery] -> Vdc 2/5  "i_battery"
  Mux4/1 -> Vdc 2/3  "i_out"
  Mux3/1 -> Vdc 2/2  "iL"
  [iL] -> Mux3/1  "iL"
  [u2] -> Mux5/2
  [V_bus] -> Vdc 2/4  "Vc"
  [i_out_ref] -> Mux4/1
  [i_out] -> Mux4/2
  From52/1 -> MATLAB Function1/6(Vc)
  [i_battery] -> Gain4/1
  [u2] -> Mux8/2
  [V_bus] -> Vdc 4/4  "V_bus"
  Mux8/1 -> Vdc 4/6  "u1,u2"
  Mux7/1 -> Vdc 4/3  "i_battery"
  [i_out] -> Gain5/1
  From62/1 -> Modulation2/2(u2)
  [u1] -> Mux8/1
  From61/1 -> Modulation2/1(u1)
  [V_battery] -> Vdc 4/1  "V_battery"
  Mux6/1 -> Vdc 4/2  "iL"
  [iL_ref] -> Mux6/2  "iL*"
  Modulation2/3(S3) -> Goto31/1
  Modulation2/4(S4) -> Goto30/1
  Modulation2/1(S1) -> Goto32/1
  Modulation2/2(S2) -> Goto29/1
  [iL] -> Gain1/1
  [i_out_ref] -> Mux7/2
  IL6/1 -> [i_battery], BatteryCurrent1/1
  From53/1 -> MATLAB Function2/5(vin)
  From74/1 -> Gain2/1
  From59/1 -> MATLAB Function2/6(Vc)
  From58/1 -> Sum2/1
  From57/1 -> MATLAB Function2/3(i_out_ref)
  PID Controller3/1 -> Goto27/1
  Sum2/1 -> PID Controller3/1
  From54/1 -> MATLAB Function2/7(Ts)
  MATLAB Function2/1(u1) -> Goto15/1
  From56/1 -> MATLAB Function2/1(iL_ref)
  MATLAB Function2/2(u2) -> Goto25/1
  From34/1 -> Gain3/1
  Constant2/1 -> Goto26/1
  From32/1 -> Gain/1
  Gain/1 -> MATLAB Function2/2(iL)
  Gain1/1 -> Mux6/1
  Gain2/1 -> Sum2/2
  Gain3/1 -> MATLAB Function2/4(i_out)
  Gain4/1 -> Mux7/1
  Gain5/1 -> Vdc 4/5  "i_bus"
  Step1/1 -> Ideal Switch/1
  Ideal Switch/1 -> Terminator4/1
  Step/1 -> Controlled Voltage Source/1
  [VC_ref] -> Mux10/2  "VC_ref"
  [iL] -> Gain8/1  "iL"
  [i_out] -> Gain9/1
  [V_battery] -> Mux10/1  "V_battery"
  Mux11/1 -> Vdc 5/6  "u1,u2"
  From88/1 -> Product3/2  "io"
  From94/1 -> Sum3/2
  [i_battery] -> Gain7/1  "i_battery"
  From80/1 -> Modulation3/1(u1)
  [iL_ref] -> Mux9/2  "iL*"
  Mux9/1 -> Vdc 5/2  "iL"
  [u2] -> Mux11/2
  [V_bus] -> Vdc 5/1  "V_bus"
  PID Controller4/1 -> Goto36/1
  From92/1 -> Product3/1  "Vc"
  [u1] -> Mux11/1
  From81/1 -> Modulation3/2(u2)
  Mux10/1 -> Vdc 5/3  "V_out"
  From75/1 -> Sum3/1
  Product3/1 -> Power3/1
  Sum3/1 -> PID Controller4/1
  Modulation3/1(S1) -> Goto41/1
  Modulation3/2(S2) -> Goto28/1
  Modulation3/3(S3) -> Goto40/1
  Modulation3/4(S4) -> Goto33/1
  Gain8/1 -> Mux9/1
  Gain9/1 -> Vdc 5/4  "i_bus"
  From95/1 -> Gain6/1
  From24/1 -> Gain10/1
  From70/1 -> MATLAB Function3/3(vc_ref)
  From76/1 -> MATLAB Function3/5(vin)
  MATLAB Function3/1(u1) -> Goto6/1
  From77/1 -> MATLAB Function3/4(vc)
  MATLAB Function3/2(u2) -> Goto7/1
  From78/1 -> MATLAB Function3/7(Ts)
  Gain6/1 -> MATLAB Function3/6(i_out)
  Gain7/1 -> Vdc 5/5  "i_battery"
  Gain10/1 -> MATLAB Function3/2(iL)
  Step2/1 -> Goto37/1
  From79/1 -> MATLAB Function3/1(iL_ref)
  VE2/1 -> V_battery 1/1
  Constant/1 -> Goto5/1
  If/5 -> If Action Subsystem/Action
  From115/1 -> Discharge + Voltage/1(V_bus)
  From116/1 -> Discharge + Voltage/2(iL)
  From117/1 -> Discharge + Voltage/3(V_battery)
  From118/1 -> Discharge + Voltage/4(I_out)
  From119/1 -> Discharge + Voltage/5(TimeStep)
  Constant6/1 -> Discharge + Voltage/6(Vc_ref)
  If/1 -> Discharge + Voltage/Action
  Charge/Discharge Mode/1 -> If/1
  Constant Voltage / Current/1 -> If/2
  Triangle Generator/1 -> Discharge + Voltage/7(Triangular_generator)
  From120/1 -> Charge + Voltage/1(V_bus)
  From123/1 -> Charge + Voltage/4(I_out)
  From124/1 -> Charge + Voltage/5(TimeStep)
  Triangle Generator1/1 -> Charge + Voltage/7(Triangular_generator)
  From121/1 -> Charge + Voltage/2(iL)
  From122/1 -> Charge + Voltage/3(V_battery)
  Constant7/1 -> Charge + Voltage/6(Vc_ref)
  If/2 -> Charge + Voltage/Action
  Discharge + Voltage/4(S4) -> Goto50/1
  Discharge + Voltage/8(u2) -> Goto54/1
  Discharge + Voltage/5(iL_ref) -> Goto52/1
  Discharge + Voltage/6(Vc_ref_show) -> Goto47/1
  Discharge + Voltage/7(u1) -> Goto53/1
  Discharge + Voltage/3(S3) -> Goto49/1
  Discharge + Voltage/1(S1) -> Goto51/1
  Discharge + Voltage/2(S2) -> Goto48/1
  S2_merge/1 -> Goto56/1
  u1_merge1/1 -> Goto61/1
  S3_merge/1 -> Goto57/1
  iL_ref_merge/1 -> Goto60/1
  u2_merge/1 -> Goto62/1
  S4_merge/1 -> Goto58/1
  S1_merge/1 -> Goto59/1
  Vc_ref_merge/1 -> Goto55/1
  Charge + Voltage/7(u1) -> Goto69/1
  Charge + Voltage/1(S1) -> Goto67/1
  Charge + Voltage/5(iL_ref) -> Goto68/1
  Charge + Voltage/2(S2) -> Goto64/1
  Charge + Voltage/4(S4) -> Goto66/1
  Charge + Voltage/6(Vc_ref_show) -> Goto63/1
  Charge + Voltage/8(u2) -> Goto70/1
  From125/1 -> S1_merge/1
  From127/1 -> S1_merge/2
  From126/1 -> S2_merge/1
  From128/1 -> S2_merge/2
  From129/1 -> S3_merge/1
  From130/1 -> S3_merge/2
  From131/1 -> S4_merge/2
  From132/1 -> S4_merge/1
  From133/1 -> iL_ref_merge/2
  From134/1 -> iL_ref_merge/1
  From135/1 -> Vc_ref_merge/2
  From136/1 -> Vc_ref_merge/1
  From137/1 -> u1_merge1/1
  From138/1 -> u1_merge1/2
  From139/1 -> u2_merge/1
  From140/1 -> u2_merge/2
  From141/1 -> Charge + Voltage/8(I_battery)
  Charge + Voltage/3(S3) -> Goto65/1
  Discharge + Current/3(S3) -> Goto73/1
  Discharge + Current/8(u2) -> Goto78/1
  Discharge + Current/4(S4) -> Goto74/1
  Discharge + Current/2(S2) -> Goto72/1
  Triangle Generator2/1 -> Discharge + Current/7(Triangular_generator)
  From145/1 -> Discharge + Current/4(I_out)
  Discharge + Current/7(u1) -> Goto77/1
  Discharge + Current/6(i_out_ref_show) -> Goto71/1
  Constant8/1 -> Discharge + Current/6(i_out_ref)
  Discharge + Current/1(S1) -> Goto75/1
  From144/1 -> Discharge + Current/3(V_battery)
  Discharge + Current/5(iL_ref) -> Goto76/1
  From146/1 -> Discharge + Current/5(TimeStep)
  From143/1 -> Discharge + Current/2(iL)
  If/3 -> Discharge + Current/Action
  From142/1 -> Discharge + Current/1(V_bus)
  From147/1 -> u2_merge/3
  From148/1 -> u1_merge1/3
  From150/1 -> iL_ref_merge/3
  From151/1 -> S4_merge/3
  From152/1 -> S3_merge/3
  From153/1 -> S2_merge/3
  From154/1 -> S1_merge/3
  From159/1 -> Charge + Current/5(TimeStep)
  From155/1 -> Charge + Current/1(V_bus)
  From156/1 -> Charge + Current/2(iL)
  Charge + Current/5(iL_ref) -> Goto85/1
  Charge + Current/3(S3) -> Goto82/1
  Charge + Current/4(S4) -> Goto83/1
  Charge + Current/1(S1) -> Goto84/1
  Charge + Current/6(i_out_ref_show) -> Goto80/1
  From160/1 -> Charge + Current/4(i_battery)
  Charge + Current/2(S2) -> Goto81/1
  Triangle Generator3/1 -> Charge + Current/7(Triangular_generator)
  Constant9/1 -> Charge + Current/6(i_out_ref)
  From157/1 -> Charge + Current/3(V_battery)
  Charge + Current/7(u1) -> Goto86/1
  Charge + Current/8(u2) -> Goto87/1
  If/4 -> Charge + Current/Action
  From149/1 -> Vc_ref_merge1/1
  Vc_ref_merge1/1 -> Goto79/1
  From158/1 -> Vc_ref_merge1/2
  From161/1 -> S1_merge/4
  From162/1 -> S2_merge/4
  From163/1 -> S3_merge/4
  From164/1 -> S4_merge/4
  From165/1 -> iL_ref_merge/4
  From166/1 -> u1_merge1/4
  From167/1 -> u2_merge/4
  [i_out_ref] -> Sum5/1
  [i_out] -> Sum5/2
  PID Controller6/1 -> [iL_ref]
  Sum5/1 -> PID Controller6/1
  Constant10/1 -> [Power_ref]
  Mux16/1 -> Vdc 3/3  "Power"
  Mux17/1 -> Vdc 3/6  "u1,u2"
  [Power_ref] -> Mux16/2
  Mux15/1 -> Vdc 3/2  "iL"
  [V_battery] -> Vdc 3/1  "V_battery"
  [iL] -> Mux15/1
  [Power_out] -> Mux16/1
  [iL_ref] -> Mux15/2  "iL*"
  [u1] -> Mux17/1
  [Power_ref] -> Divide/1
  [V_bus] -> Product4/1, Divide/2
  Divide/1 -> [i_out_ref]
  [i_out] -> Product4/2
  Product4/1 -> ActualPower/1, [Power_out]
  [iL_ref] -> MATLAB Function5/1(iL_ref)
  MATLAB Function5/2(u2) -> [u2]
  [u1] -> Modulation5/1(u1)
  [i_out_ref] -> MATLAB Function5/3(i_out_ref)
  [i_out] -> MATLAB Function5/4(i_out)
  Modulation5/1(S1) -> [S1]
  MATLAB Function5/1(u1) -> [u1]
  [u2] -> Modulation5/2(u2)
  [V_battery] -> MATLAB Function5/5(vin)
  Modulation5/2(S2) -> [S2]
  [iL] -> MATLAB Function5/2(iL)
  [Ts] -> MATLAB Function5/7(Ts)
  Modulation5/4(S4) -> [S4]
  Modulation5/3(S3) -> [S3]
  [V_bus] -> MATLAB Function5/6(Vc)
  Constant11/1 -> [V_power_starup]
  [V_bus] -> Mux18/1  "V_bus"
  Mux18/1 -> Vdc 3/4  "V_out"
  [V_power_starup] -> Mux18/2
  [i_out] -> Mux19/1  "i_bus"
  [i_out_ref] -> Mux19/2  "i_ref"
  Mux19/1 -> Vdc 3/5  "i_out"
  [u2] -> Mux17/2
  connections:
  "85 volts, 100 Ah LithiumIon battery "/LConn2 -- VE2/LConn2 -- R_battery/LConn1
  IGBT/Diode1/RConn1 -- mid_R/RConn1 -- IGBT/Diode2/LConn1
  IGBT/Diode4/LConn1 -- Current Measurement/RConn1 -- IGBT/Diode3/RConn1
  mid_L/RConn1 -- Current Measurement/LConn1
  mid_R/LConn1 -- mid_L/LConn1
  Current Measurement1/RConn1 -- +/RConn1
  IL6/LConn1 -- Controlled Voltage Source/RConn1 -- Ideal Switch/RConn1 -- VE2/LConn1 -- "85 volts, 100 Ah LithiumIon battery "/LConn1
  VE/LConn1 -- IL6/RConn1 -- C1/LConn1 -- IGBT/Diode1/LConn1
  C1/RConn1 -- "init_bat  "/LConn1 -- R_battery/RConn1 -- Controlled Voltage Source/LConn1 -- VE1/LConn2 -- C2/RConn1 -- -/RConn1 -- IGBT/Diode4/RConn1 -- IGBT/Diode2/RConn1 -- VE/LConn2
  Ideal Switch/LConn1 -- "init_bat  "/RConn1
  C2/LConn1 -- VE1/LConn1 -- Current Measurement1/LConn1 -- IGBT/Diode3/LConn1

== system Battery_charge_discharge_FSBB_DCDC/InitSystem ==

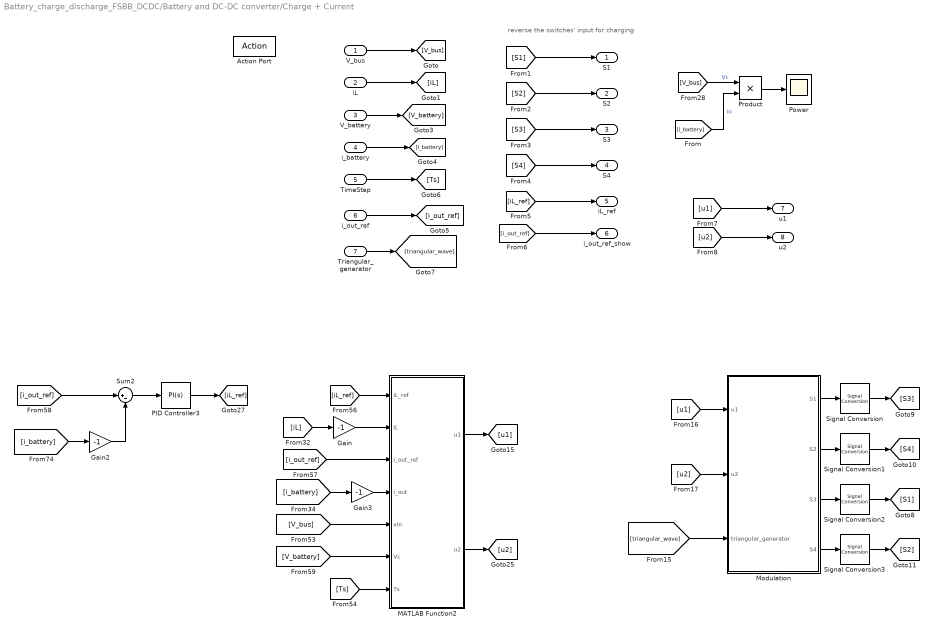
== system Battery_charge_discharge_FSBB_DCDC/Battery and DC-DC converter/Charge + Current ==
  note: reverse the switches' input for charging
  V_bus : Inport
  iL : Inport  Port=2
  V_battery : Inport  Port=3
  i_battery : Inport  Port=4
  TimeStep : Inport  Port=5
  i_out_ref : Inport  Port=6
  Triangular_generator : Inport  Port=7
  Action Port : ActionPort  ActionPortLabel=elseif( u1==0 & u2==1)
  Gain : Gain  Gain=-1
  Gain2 : Gain  Gain=-1
  Gain3 : Gain  Gain=-1
  MATLAB Function2 : MATLAB Function  TreatAsAtomicUnit=on
  Modulation : Subsystem
  PID Controller3 : slpidlib/PID Controller  Controller=PI  Form=Parallel  TimeDomain=Continuous-time  UseExternalTs=off  SampleTime=-1  IntegratorMethod=Forward Euler  FilterMethod=Forward Euler  ControllerParametersSource=internal  P=15  I=1000  UseKiTs=on  D=0  N=100  UseFilter=on  TunerSelectOption=Transfer Function Based (PID Tuner App)  InitialConditionSource=internal  InitialConditionForIntegrator=0  InitialConditionForFilter=0  DifferentiatorICPrevScaledInput=0  ExternalReset=none  TrackingMode=off  Kt=1  LimitOutput=on  SatLimitsSource=internal  UpperSaturationLimit=50  LowerSaturationLimit=-10  LinearizeAsGain=on  AntiWindupMode=none  Kb=1  LimitIntegrator=off  UpperIntegratorSaturationLimit=inf  LowerIntegratorSaturationLimit=-inf  POutMin=[]  POutMax=[]  IOutMin=[]  IOutMax=[]  DOutMin=[]  DOutMax=[]  NOutMin=[]  NOutMax=[]  SumOutMin=[]  SumOutMax=[]  SaturationOutMin=[]  SaturationOutMax=[]  PParamMin=[]  PParamMax=[]  IParamMin=[]  IParamMax=[]  DParamMin=[]  DParamMax=[]  NParamMin=[]  NParamMax=[]  KbParamMin=[]  KbParamMax=[]  KtParamMin=[]  KtParamMax=[]  KbOutMin=[]  KbOutMax=[]  KtOutMin=[]  KtOutMax=[]  IntegratorOutMin=[]  IntegratorOutMax=[]  FilterOutMin=[]  FilterOutMax=[]  SumI1OutMin=[]  SumI1OutMax=[]  SumI2OutMin=[]  SumI2OutMax=[]  SumI3OutMin=[]  SumI3OutMax=[]  SumI4OutMin=[]  SumI4OutMax=[]  SumDOutMin=[]  SumDOutMax=[]  DifferentiatorOutMin=[]  DifferentiatorOutMax=[]  FilterDiffOutCoefMin=[]  FilterDiffOutCoefMax=[]  ReciprocalOutMin=[]  ReciprocalOutMax=[]  SumDenOutMin=[]  SumDenOutMax=[]  SumNumOutMin=[]  SumNumOutMax=[]  DivideOutMin=[]  DivideOutMax=[]  UdiffTsProdOutMin=[]  UdiffTsProdOutMax=[]  NTsProdOutMin=[]  NTsProdOutMax=[]  UintegralTsProdOutMin=[]  UintegralTsProdOutMax=[]  UngainTsProdOutMin=[]  UngainTsProdOutMax=[]  ClampingZeroOutDataTypeStr=Inherit: Inherit via back propagation  ClampingZeroOutMin=[]  ClampingZeroOutMax=[]  FilterDenConstantOutDataTypeStr=Inherit: Inherit via back propagation  FilterDenConstantOutMin=[]  FilterDenConstantOutMax=[]  PCopyOutDataTypeStr=Inherit: Inherit via back propagation  PCopyOutMin=[]  PCopyOutMax=[]  NCopyOutDataTypeStr=Inherit: Inherit via back propagation  NCopyOutMin=[]  NCopyOutMax=[]  IntegratorContinuousStateAttributes=''  IntegratorStateMustResolveToSignalObject=off  IntegratorRTWStateStorageClass=Auto  FilterContinuousStateAttributes=''  FilterStateMustResolveToSignalObject=off  FilterRTWStateStorageClass=Auto  ParallelPVariant=InternalParameters  IdealPVariant=Disabled  IVariant=InternalParameters  DVariant=Disabled  IntegratorVariant=Continuous  SatVariant=Enabled  AWVariant=Passthrough  PCopyVariant=Disabled  TRVariant=Disabled  FdbkBlocksVariant=Forward  IdealPFdbkVariant=Disabled  SatFdbkVariant=Disabled  DerivativeFilterVariant=Disabled  NVariant=Disabled  NCopyVariant=Disabled_SignalSpec  FilterICVariant=Disabled  IntegratorICVariant=InternalICs  ExternalResetVariant=Disabled  TRSumVariant=Passthrough  SumFdbkVariant=Disabled  SumVariant=Sum_PI  TsampFilterVariant=InternalTs  TsampNgainVariant=Passthrough  TsampIntegralVariant=Passthrough  ExternalSaturationOutDataTypeStr=Inherit: Same as second input
  Power : Scope
  Product : Product
  Signal Conversion{,1..3} (4 alike) : SignalConversion  OverrideOpt=off
  Sum2 : Sum  Inputs=|+-
  S1 : Outport
  S2 : Outport  Port=2
  S3 : Outport  Port=3
  S4 : Outport  Port=4
  iL_ref : Outport  Port=5
  i_out_ref_show : Outport  Port=6
  u1 : Outport  Port=7
  u2 : Outport  Port=8
  wires:
  Modulation/2(S2) -> Signal Conversion1/1
  Modulation/1(S1) -> Signal Conversion/1
  Modulation/3(S3) -> Signal Conversion2/1
  [u1] -> Modulation/1(u1)
  [i_battery] -> Product/2  "io"
  [u2] -> Modulation/2(u2)
  [V_bus] -> Product/1  "Vc"
  Product/1 -> Power/1
  Modulation/4(S4) -> Signal Conversion3/1
  V_bus/1 -> [V_bus]
  iL/1 -> [iL]
  V_battery/1 -> [V_battery]
  i_battery/1 -> [i_battery]
  TimeStep/1 -> [Ts]
  i_out_ref/1 -> [i_out_ref]
  [iL_ref] -> iL_ref/1
  [i_out_ref] -> i_out_ref_show/1
  [u2] -> u2/1
  [u1] -> u1/1
  [triangular_wave] -> Modulation/3(triangular_generator)
  Triangular_generator/1 -> [triangular_wave]
  [S1] -> S1/1
  [S3] -> S3/1
  [S4] -> S4/1
  [S2] -> S2/1
  [i_out_ref] -> Sum2/1
  [i_battery] -> Gain3/1
  MATLAB Function2/1(u1) -> [u1]
  [iL] -> Gain/1
  Gain/1 -> MATLAB Function2/2(iL)
  Gain2/1 -> Sum2/2
  [V_bus] -> MATLAB Function2/5(vin)
  Gain3/1 -> MATLAB Function2/4(i_out)
  MATLAB Function2/2(u2) -> [u2]
  [iL_ref] -> MATLAB Function2/1(iL_ref)
  PID Controller3/1 -> [iL_ref]
  [Ts] -> MATLAB Function2/7(Ts)
  [i_battery] -> Gain2/1
  Sum2/1 -> PID Controller3/1
  [i_out_ref] -> MATLAB Function2/3(i_out_ref)
  [V_battery] -> MATLAB Function2/6(Vc)
  Signal Conversion1/1 -> [S4]
  Signal Conversion/1 -> [S3]
  Signal Conversion2/1 -> [S1]
  Signal Conversion3/1 -> [S2]

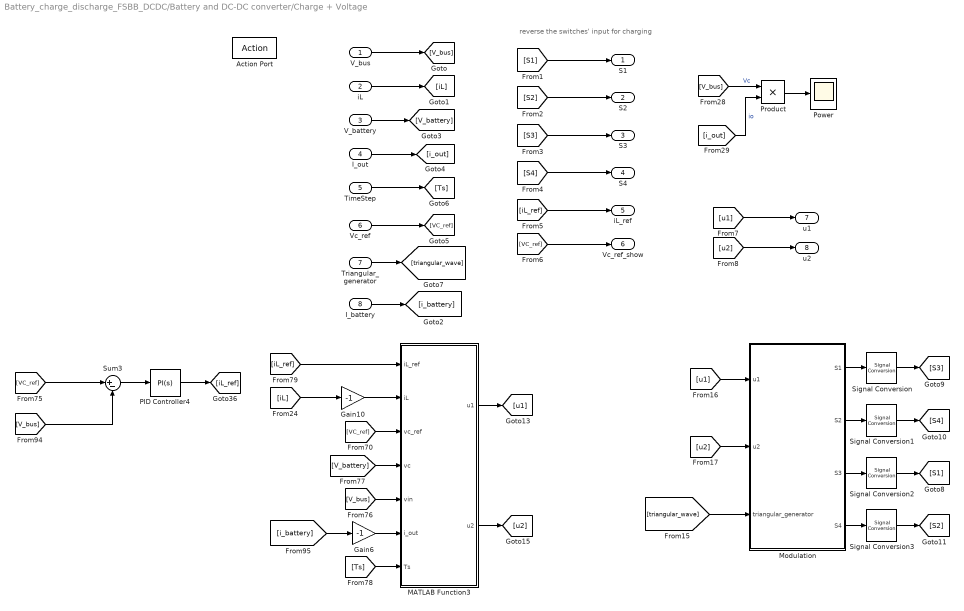
== system Battery_charge_discharge_FSBB_DCDC/Battery and DC-DC converter/Charge + Voltage ==
  note: reverse the switches' input for charging
  V_bus : Inport
  iL : Inport  Port=2
  V_battery : Inport  Port=3
  I_out : Inport  Port=4
  TimeStep : Inport  Port=5
  Vc_ref : Inport  Port=6
  Triangular_generator : Inport  Port=7
  I_battery : Inport  Port=8
  Action Port : ActionPort  ActionPortLabel=elseif(u1 == 0 & u2 ==0)
  Gain10 : Gain  Gain=-1
  Gain6 : Gain  Gain=-1
  MATLAB Function3 : MATLAB Function  TreatAsAtomicUnit=on
  Modulation : Subsystem
  PID Controller4 : slpidlib/PID Controller  Controller=PI  Form=Parallel  TimeDomain=Continuous-time  UseExternalTs=off  SampleTime=-1  IntegratorMethod=Forward Euler  FilterMethod=Forward Euler  ControllerParametersSource=internal  P=15  I=1000  UseKiTs=on  D=0  N=100  UseFilter=on  TunerSelectOption=Transfer Function Based (PID Tuner App)  InitialConditionSource=internal  InitialConditionForIntegrator=0  InitialConditionForFilter=0  DifferentiatorICPrevScaledInput=0  ExternalReset=none  TrackingMode=off  Kt=1  LimitOutput=on  SatLimitsSource=internal  UpperSaturationLimit=50  LowerSaturationLimit=-10  LinearizeAsGain=on  AntiWindupMode=none  Kb=1  LimitIntegrator=off  UpperIntegratorSaturationLimit=inf  LowerIntegratorSaturationLimit=-inf  POutMin=[]  POutMax=[]  IOutMin=[]  IOutMax=[]  DOutMin=[]  DOutMax=[]  NOutMin=[]  NOutMax=[]  SumOutMin=[]  SumOutMax=[]  SaturationOutMin=[]  SaturationOutMax=[]  PParamMin=[]  PParamMax=[]  IParamMin=[]  IParamMax=[]  DParamMin=[]  DParamMax=[]  NParamMin=[]  NParamMax=[]  KbParamMin=[]  KbParamMax=[]  KtParamMin=[]  KtParamMax=[]  KbOutMin=[]  KbOutMax=[]  KtOutMin=[]  KtOutMax=[]  IntegratorOutMin=[]  IntegratorOutMax=[]  FilterOutMin=[]  FilterOutMax=[]  SumI1OutMin=[]  SumI1OutMax=[]  SumI2OutMin=[]  SumI2OutMax=[]  SumI3OutMin=[]  SumI3OutMax=[]  SumI4OutMin=[]  SumI4OutMax=[]  SumDOutMin=[]  SumDOutMax=[]  DifferentiatorOutMin=[]  DifferentiatorOutMax=[]  FilterDiffOutCoefMin=[]  FilterDiffOutCoefMax=[]  ReciprocalOutMin=[]  ReciprocalOutMax=[]  SumDenOutMin=[]  SumDenOutMax=[]  SumNumOutMin=[]  SumNumOutMax=[]  DivideOutMin=[]  DivideOutMax=[]  UdiffTsProdOutMin=[]  UdiffTsProdOutMax=[]  NTsProdOutMin=[]  NTsProdOutMax=[]  UintegralTsProdOutMin=[]  UintegralTsProdOutMax=[]  UngainTsProdOutMin=[]  UngainTsProdOutMax=[]  ClampingZeroOutDataTypeStr=Inherit: Inherit via back propagation  ClampingZeroOutMin=[]  ClampingZeroOutMax=[]  FilterDenConstantOutDataTypeStr=Inherit: Inherit via back propagation  FilterDenConstantOutMin=[]  FilterDenConstantOutMax=[]  PCopyOutDataTypeStr=Inherit: Inherit via back propagation  PCopyOutMin=[]  PCopyOutMax=[]  NCopyOutDataTypeStr=Inherit: Inherit via back propagation  NCopyOutMin=[]  NCopyOutMax=[]  IntegratorContinuousStateAttributes=''  IntegratorStateMustResolveToSignalObject=off  IntegratorRTWStateStorageClass=Auto  FilterContinuousStateAttributes=''  FilterStateMustResolveToSignalObject=off  FilterRTWStateStorageClass=Auto  ParallelPVariant=InternalParameters  IdealPVariant=Disabled  IVariant=InternalParameters  DVariant=Disabled  IntegratorVariant=Continuous  SatVariant=Enabled  AWVariant=Passthrough  PCopyVariant=Disabled  TRVariant=Disabled  FdbkBlocksVariant=Forward  IdealPFdbkVariant=Disabled  SatFdbkVariant=Disabled  DerivativeFilterVariant=Disabled  NVariant=Disabled  NCopyVariant=Disabled_SignalSpec  FilterICVariant=Disabled  IntegratorICVariant=InternalICs  ExternalResetVariant=Disabled  TRSumVariant=Passthrough  SumFdbkVariant=Disabled  SumVariant=Sum_PI  TsampFilterVariant=InternalTs  TsampNgainVariant=Passthrough  TsampIntegralVariant=Passthrough  ExternalSaturationOutDataTypeStr=Inherit: Same as second input
  Power : Scope
  Product : Product
  Signal Conversion{,1..3} (4 alike) : SignalConversion  OverrideOpt=off
  Sum3 : Sum  Inputs=|+-
  S1 : Outport
  S2 : Outport  Port=2
  S3 : Outport  Port=3
  S4 : Outport  Port=4
  iL_ref : Outport  Port=5
  Vc_ref_show : Outport  Port=6
  u1 : Outport  Port=7
  u2 : Outport  Port=8
  wires:
  Modulation/2(S2) -> Signal Conversion1/1
  Modulation/1(S1) -> Signal Conversion/1
  Modulation/3(S3) -> Signal Conversion2/1
  [u1] -> Modulation/1(u1)
  [i_out] -> Product/2  "io"
  [u2] -> Modulation/2(u2)
  [V_bus] -> Product/1  "Vc"
  Product/1 -> Power/1
  Modulation/4(S4) -> Signal Conversion3/1
  V_bus/1 -> [V_bus]
  iL/1 -> [iL]
  V_battery/1 -> [V_battery]
  I_out/1 -> [i_out]
  TimeStep/1 -> [Ts]
  Vc_ref/1 -> [VC_ref]
  [iL_ref] -> iL_ref/1
  [VC_ref] -> Vc_ref_show/1
  [u2] -> u2/1
  [u1] -> u1/1
  [triangular_wave] -> Modulation/3(triangular_generator)
  Triangular_generator/1 -> [triangular_wave]
  Sum3/1 -> PID Controller4/1
  [VC_ref] -> MATLAB Function3/3(vc_ref)
  Gain10/1 -> MATLAB Function3/2(iL)
  [iL] -> Gain10/1
  [V_bus] -> MATLAB Function3/5(vin)
  MATLAB Function3/2(u2) -> [u2]
  Gain6/1 -> MATLAB Function3/6(i_out)
  [V_bus] -> Sum3/2
  [iL_ref] -> MATLAB Function3/1(iL_ref)
  [Ts] -> MATLAB Function3/7(Ts)
  MATLAB Function3/1(u1) -> [u1]
  [VC_ref] -> Sum3/1
  [V_battery] -> MATLAB Function3/4(vc)
  [i_battery] -> Gain6/1
  PID Controller4/1 -> [iL_ref]
  I_battery/1 -> [i_battery]
  Signal Conversion/1 -> [S3]
  Signal Conversion1/1 -> [S4]
  Signal Conversion3/1 -> [S2]
  Signal Conversion2/1 -> [S1]
  [S2] -> S2/1
  [S1] -> S1/1
  [S3] -> S3/1
  [S4] -> S4/1
